simulink model "env_sim"  (R2015b)
settings: Solver=FixedStepAuto  StartTime=0.0  StopTime=20.0  FixedStep=0.001  RelTol=1e-3
values from neighbouring files (symbols this model uses):
  CG_dry = [0 0 0]    [Sim_Script.m]
  CG_e = [0 0 -1.0]    [Sim_Script.m]
  m_dry = 10    [Sim_Script.m]
  m_f = (31.8)./1000    [Sim_Script.m]
  m_o = M_t - m_f    [Sim_Script.m]
  TC = dlmread('AeroTech_F30.eng',' ',2,3)    [Sim_Script.m]
  TI = 47.0    (= 47)    [Sim_Script.m]
libraries: realtime_pacer_lib x2
settings Model: Creator=Mitchel  LastModifiedBy=Mitchel

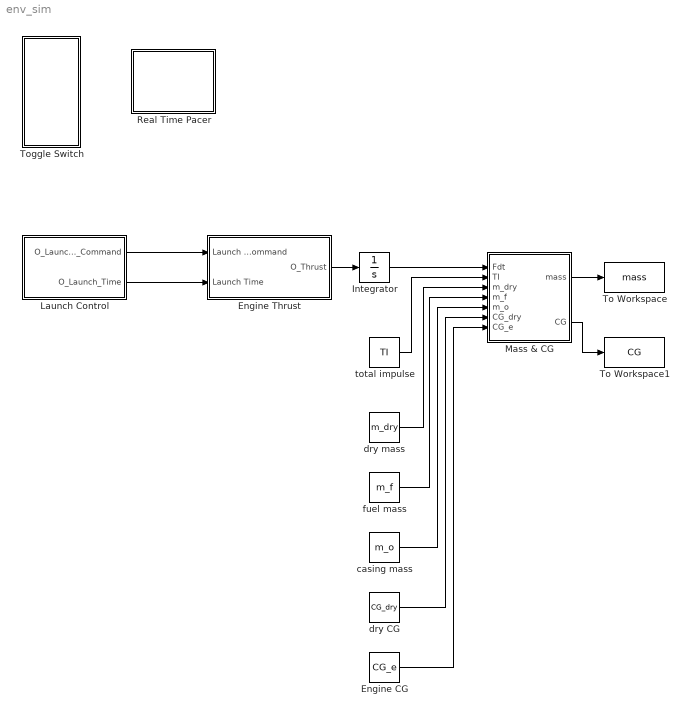
== system env_sim ==
  Engine CG : Constant  Value=CG_e
  "Engine Thrust " : Subsystem
  Integrator : Integrator
  Launch Control : Subsystem
  "Mass & CG " : MATLAB Function  TreatAsAtomicUnit=on
  "Real Time Pacer " : Subsystem
  To Workspace : ToWorkspace  VariableName=mass  SampleTime=-1
  To Workspace1 : ToWorkspace  VariableName=CG  SampleTime=-1
  Toggle Switch : Subsystem  DialogController=hmiCreateDDGDialog  IsWebBlock=on  mask(MWDashboardBlock){webBlockId=36622ab1-1db6-4c19-9be9-f562fd1bb84c, webBlockType=toggleswitch, ShowInLibBrowser=on, ShowInitialText=on, HMISrcModelName=env_sim}
      mask prompts: webBlockId "WebBlock Id"; webBlockType "WebBlock Type"; HMISrcModelName "Source Model"
      mask Help: helpview([docroot '/mapfiles/simulink.map'], 'hmi_toggle_switch')
      mask Display:
      | if strcmp(get_param(bdroot(gcb),'BlockDiagramType'), 'library')
      |     image([(matlabroot) '/toolbox/simulink/hmi/icons/ToggleSwitch.png']);
      | end
  casing mass : Constant  Value=m_o
  dry CG : Constant  Value=CG_dry
  "dry mass " : Constant  Value=m_dry
  fuel mass : Constant  Value=m_f
  total impulse : Constant  Value=TI
  wires:
  Launch Control/1(O_Launch_Command) -> "Engine Thrust "/1(Launch Command)
  Launch Control/2(O_Launch_Time) -> "Engine Thrust "/2("Launch Time ")
  "Engine Thrust "/1(O_Thrust) -> Integrator/1
  Integrator/1 -> "Mass & CG "/1(Fdt)
  total impulse/1 -> "Mass & CG "/2(TI)
  "dry mass "/1 -> "Mass & CG "/3(m_dry)
  fuel mass/1 -> "Mass & CG "/4(m_f)
  casing mass/1 -> "Mass & CG "/5(m_o)
  dry CG/1 -> "Mass & CG "/6(CG_dry)
  Engine CG/1 -> "Mass & CG "/7(CG_e)
  "Mass & CG "/1(mass) -> To Workspace/1
  "Mass & CG "/2(CG) -> To Workspace1/1

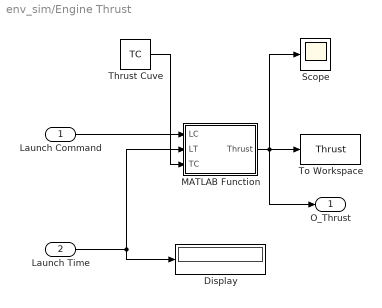
== system env_sim/Engine Thrust  ==
  Launch Command : Inport
  "Launch Time " : Inport  Port=2
  Display : Display
  MATLAB Function : MATLAB Function  TreatAsAtomicUnit=on
  Scope : Scope
  Thrust Cuve : Constant  Value=TC
  To Workspace : ToWorkspace  VariableName=Thrust  SaveFormat=Timeseries  SampleTime=-1
  O_Thrust : Outport
  wires:
  MATLAB Function/1(Thrust) -> O_Thrust/1, Scope/1, To Workspace/1
  Thrust Cuve/1 -> MATLAB Function/3(TC)
  Launch Command/1 -> MATLAB Function/1(LC)
  "Launch Time "/1 -> MATLAB Function/2(LT), Display/1

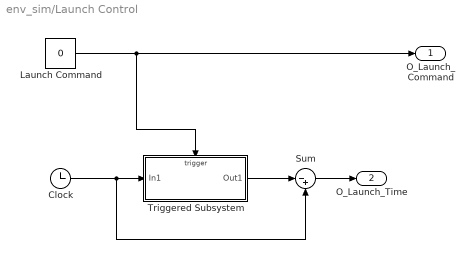
== system env_sim/Launch Control ==
  Clock : Clock
  Launch Command : Constant  Value=0
  Sum : Sum  Inputs=|-+
  Triggered Subsystem : Subsystem  TreatAsAtomicUnit=on
  O_Launch_Command : Outport
  O_Launch_Time : Outport  Port=2
  wires:
  Launch Command/1 -> O_Launch_Command/1, Triggered Subsystem/Trigger
  Clock/1 -> Triggered Subsystem/1(In1), Sum/2
  Sum/1 -> O_Launch_Time/1
  Triggered Subsystem/1(Out1) -> Sum/1

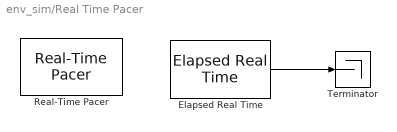
== system env_sim/Real Time Pacer  ==
  Elapsed Real Time : realtime_pacer_lib/Elapsed Real Time
  Real-Time Pacer : realtime_pacer_lib/Real-Time Pacer  simTimePerRealTime=1
  Terminator : Terminator
  wires:
  Elapsed Real Time/1 -> Terminator/1

== system env_sim/Toggle Switch ==

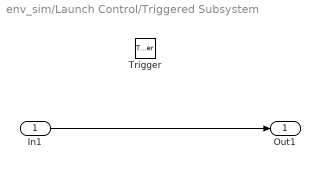
== system env_sim/Launch Control/Triggered Subsystem ==
  In1 : Inport
  Trigger : TriggerPort
  Out1 : Outport
  wires:
  In1/1 -> Out1/1

== matlab function env_sim/Mass & CG  ==
  data: Fdt input; TI input; mass output; m_dry input; m_f input; m_o input; CG_dry input; CG_e input; CG output
function [mass,CG] = fcn(Fdt,TI,m_dry, m_f, m_o, CG_dry, CG_e)
%Mass and CG calculator

%Engine mass at time t:
me_t = m_o + m_f.*(1-(1./TI).*(Fdt))

mass = me_t + m_dry;

%CG calculation:
CG =  (me_t.*CG_e+m_dry.*CG_dry)./(mass)

== matlab function env_sim/Engine Thrust /MATLAB Function ==
  data: LC input; Thrust output; LT input; TC input
function Thrust = fcn(LC,LT, TC)
% Thrust Curve Interpolator
TC_t = TC(:,1);
TC_f = TC(:,2);

Thrust = 0;

%Check to see if a launch command has been sent.
if LC>0
    Thrust = interp1(TC_t,TC_f,LT); %Find interpolated thrust value from launch time, in Newtons.
    
    %if at end of time.
    if isnan(Thrust)
        Thrust = 0;
    end
    Thrust
end
